simulink model "GFL_GFM"  (R2024b)
settings: Solver=FixedStepAuto  StartTime=0.0  StopTime=1.2  FixedStep=1E-6  RelTol=1e-3
InitFcn:
  | %电网阻抗参数-------------------------------
  | Rg=0.000008; Lg=0.4e-3;
  | Sn=2000000;
  | k=0.6;
  | %分配比例,在这里设置分配比例，GFL：GFM=k:(1-k)
  | PGFL=Sn*k;PGFM=Sn*(1-k);
  | 
  | %GFL参数------------------------------------
  | L_GFL=70e-6;  C_GFL=80e-6; R_GFL=0.2;
  | R1=0;L1=2e-4;
  | Ppll=0.8;Ipll=200;
  | Pp_GFL=0.001;Ip_GFL=0.14;
  | %电流环参数
  | Pp=0.0002;Ip=0.06;Max=2000;
  | Pp2=0.0002;Ip2=0.0008;Max2=200;
  | Pi_GFL=5;Ii_GFL=500;
  | 
  | %GFM参数------------------------------------
  | L_GFM=35e-6; R_GFM=0; C_GFM=150e-6;
  | R2=0;L2=1e-4;
  | %功率环
  | J=7.8; D=1200; Kf=300;
  | Kv=200; Ku=120;
  | %电压电流内环
  | Pv_GFM=66;Iv_GFM=800;
  | Pi_GFM=10;Ii_GFM=100;
model workspace (MAT data in the model file):
  uniqueStringPll_745 = '81_4724'
libraries: spsSeriesRLCBranchLib x12, slpidlib x11, spsabctodq0Lib x7, spsThreePhaseVIMeasurementLib x4, spsGroundLib x3, spsThreePhaseSeriesRLCBranchLib x3, spsThreePhaseTransformerTwoWindingsLib x3, spsDCVoltageSourceLib x2, spsPWMGenerator3LevelLib x2, spsdq0toabcLib x2, spsThreeLevelBridgeLib x2, spsPLL3phLib x1
(part 1 of 2)
settings Model: Creator=Simulink  LastModifiedBy=SESA504213
settings SolverCC: AlgebraicLoopSolver=TrustRegion
settings DataIOCC: ReturnWorkspaceOutputs=off
settings DebuggingCC: UnconnectedInputMsg=warning  UnconnectedOutputMsg=warning  UnconnectedLineMsg=warning  ArithmeticOperatorsInVariantConditions=warning
settings ModelReferenceCC: EnableRefExpFcnMdlSchedulingChecks=on
settings SFSimCC: CustomCodeUndefinedFunction=UseInterfaceOnly
settings RTWCC: GPUComputeCapability=3.5
settings SimscapeCC: SimscapeLogType=all  SimscapeLogLimitData=off

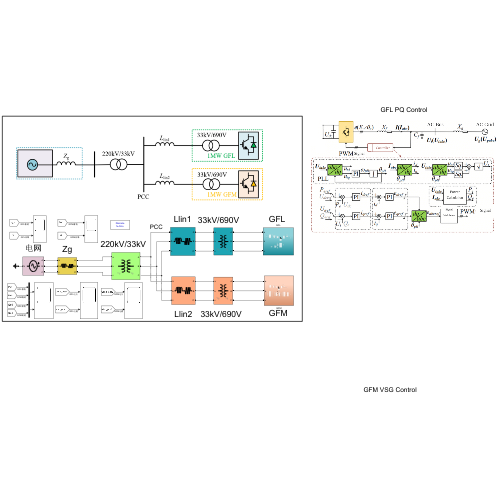
[thumbnail: Simulink's stored preview of the top-level diagram]
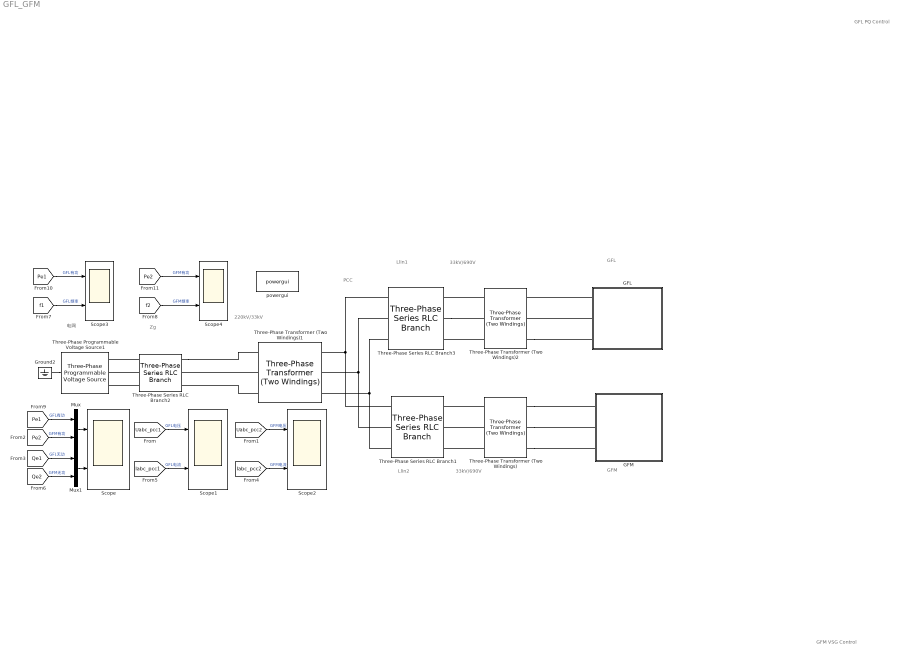
== system GFL_GFM ==
  note: GFL PQ Control
  note: Llin1
  note: PCC
  note: 220kV/33kV
  note: 电网
  note: Zg
  note: Llin2
  note: 33kV/690V
  note: 33kV/690V
  note: GFL
  note: GFM
  note: GFM VSG Control
  GFL : Subsystem
  GFM : Subsystem
  Ground2 : spsGroundLib/Ground  LConnTagsString=a
  Mux : Mux  Inputs=2
  Mux1 : Mux  Inputs=2
  Scope{,1..4} (5 alike) : Scope  NumInputPorts=2
  Three-Phase Programmable Voltage Source1 : spsThreePhaseProgrammableVoltageSourceLib/Three-Phase Programmable Voltage Source  PositiveSequence=[220e3 0 50]  VariationEntity=Frequency  VariationType=Step  VariationTypeAlt=Step  VariationStep=-0.1  VariationRate=10  VariationMagnitude=0.3  VariationFrequency=2  VariationTiming=[0.4 0.8]  VariationPhaseA=off  Amplitudes=[1 0.8 1.2 1.0]  TimeValues=[0 0.1 0.15 0.2]  HarmonicGeneration=off  HarmonicA=[3 0.2 -25 0]  HarmonicB=[2 0.15 35 2]  Timing="[0.05  3]"  BusType=swing  Pref=0  Qref=0  Qmin=-inf  Qmax=inf
  Three-Phase Series RLC Branch1 : spsThreePhaseSeriesRLCBranchLib/Three-Phase Series RLC Branch  LConnTagsString=A|B|C  RConnTagsString=A|B|C  BranchType=RL  Resistance=R2  Inductance=L2  Capacitance=1e-6  Measurements=None
  Three-Phase Series RLC Branch2 : spsThreePhaseSeriesRLCBranchLib/Three-Phase Series RLC Branch  LConnTagsString=A|B|C  RConnTagsString=A|B|C  BranchType=RL  Resistance=Rg*(10e3/690)*(10e3/690)  Inductance=Lg*(10e3/690)*(10e3/690)  Capacitance=1e-6  Measurements=None
  Three-Phase Series RLC Branch3 : spsThreePhaseSeriesRLCBranchLib/Three-Phase Series RLC Branch  LConnTagsString=A|B|C  RConnTagsString=A|B|C  BranchType=RL  Resistance=R1  Inductance=L1  Capacitance=1e-6  Measurements=None
  Three-Phase Transformer (Two Windings) : spsThreePhaseTransformerTwoWindingsLib/Three-Phase Transformer (Two Windings)  Winding1Connection=Yg  Winding2Connection=Yg  CoreType=Three single-phase transformers  SetSaturation=off  Hysteresis=off  DataFile='hysteresis'  SetInitialFlux=off  Measurements=None  UNITS=pu  NominalPower=[ 5e6 , 50 ]  Winding1=[ 690 , 0.002 , 0.08 ]  Winding2=[ 33e3 , 0.002 , 0.08 ]  Rm=500  Lm=500  L0=0.5  Saturation=[ 0,0 ; 0.0024,1.2 ; 1.0,1.52 ]  InitialFluxes=[ 0.8 , -0.8 , 0.7 ]  BreakLoop=off  DiscreteSolver=Trapezoidal iterative  DataType=off  TransfoNumber=1
  Three-Phase Transformer (Two Windings)1 : spsThreePhaseTransformerTwoWindingsLib/Three-Phase Transformer (Two Windings)  Winding1Connection=Yg  Winding2Connection=Yg  CoreType=Three single-phase transformers  SetSaturation=off  Hysteresis=off  DataFile='hysteresis'  SetInitialFlux=off  Measurements=None  UNITS=pu  NominalPower=[ 5e6 , 50 ]  Winding1=[ 33e3 , 0.002 , 0.08 ]  Winding2=[ 220e3 , 0.002 , 0.08 ]  Rm=500  Lm=500  L0=0.5  Saturation=[ 0,0 ; 0.0024,1.2 ; 1.0,1.52 ]  InitialFluxes=[ 0.8 , -0.8 , 0.7 ]  BreakLoop=off  DiscreteSolver=Trapezoidal iterative  DataType=off  TransfoNumber=1
  Three-Phase Transformer (Two Windings)2 : spsThreePhaseTransformerTwoWindingsLib/Three-Phase Transformer (Two Windings)  Winding1Connection=Yg  Winding2Connection=Yg  CoreType=Three single-phase transformers  SetSaturation=off  Hysteresis=off  DataFile='hysteresis'  SetInitialFlux=off  Measurements=None  UNITS=pu  NominalPower=[ 5e6 , 60 ]  Winding1=[ 690 , 0.002 , 0.08 ]  Winding2=[33e3 , 0.002 , 0.08 ]  Rm=500  Lm=500  L0=0.5  Saturation=[ 0,0 ; 0.0024,1.2 ; 1.0,1.52 ]  InitialFluxes=[ 0.8 , -0.8 , 0.7 ]  BreakLoop=off  DiscreteSolver=Trapezoidal iterative  DataType=off  TransfoNumber=1
  powergui : spspowerguiLib/powergui  Priority=1  SimulationMode=Discrete  SampleTime=1E-6  frequency=60  Iterations=50  frequencyindice=0  Pbase=100e6  ErrMax=1e-4  UnitsV=kV  UnitsW=MW  buscounter=0  FunctionMessages=off  echomessages=off  EnableUseOfTLC=off  CurrentSourceSwitches=off  DisableSnubberDevices=off  DisableRonSwitches=off  DisableVfSwitches=off  DisplayEquations=off  AutomaticDiscreteSolvers=off  SolverType=Tustin/Backward Euler (TBE)  Interpol=off  ExternalGateDelay=off  methode=off  Ts=100  x0status=blocks  SPID=off  SwTol=0  HookPort=off  NonlinearTolerance=1e-4  nMaxIteration=100  ContinueOnMaxIteration=off  RestoreLinks=warning  ResistiveCurrentMeasurement=off  Frange=[0:2:500]  Ylog=off  Xlog=on  ShowGrid=off  save=off  variable=ZData  structure=ScopeData1  ZoomFFT=off  StartTime=0.0  cycles=1  DisplayStyle=1  fundamental=60  FreqAxis=off  MaxFrequency=1000  frequencyindicesteady=1  RmsSteady=1  display=off
  wires:
  [Qe1] -> Mux1/1  "GFL无功"
  [Qe2] -> Mux1/2  "GFM无功"
  Mux/1 -> Scope/1
  [Pe2] -> Mux/2  "GFM有功"
  Mux1/1 -> Scope/2
  [Pe1] -> Mux/1  "GFL有功"
  [Uabc_pcc1] -> Scope1/1  "GFL电压"
  [Iabc_pcc1] -> Scope1/2  "GFL电流"
  [Uabc_pcc2] -> Scope2/1  "GFM电压"
  [Iabc_pcc2] -> Scope2/2  "GFM电流"
  [Pe1] -> Scope3/1  "GFL有功"
  [f1] -> Scope3/2  "GFL频率"
  [Pe2] -> Scope4/1  "GFM有功"
  [f2] -> Scope4/2  "GFM频率"
  connections:
  Three-Phase Transformer (Two Windings)/RConn3 -- Three-Phase Series RLC Branch1/LConn3
  Three-Phase Transformer (Two Windings)/RConn1 -- Three-Phase Series RLC Branch1/LConn1
  Three-Phase Transformer (Two Windings)/RConn2 -- Three-Phase Series RLC Branch1/LConn2
  Ground2/LConn1 -- Three-Phase Programmable Voltage Source1/LConn1
  Three-Phase Transformer (Two Windings)/LConn1 -- GFM/RConn1
  Three-Phase Transformer (Two Windings)/LConn2 -- GFM/RConn2
  Three-Phase Transformer (Two Windings)/LConn3 -- GFM/RConn3
  Three-Phase Series RLC Branch3/RConn2 -- Three-Phase Series RLC Branch1/RConn2 -- Three-Phase Transformer (Two Windings)1/LConn2
  Three-Phase Series RLC Branch3/RConn1 -- Three-Phase Series RLC Branch1/RConn1 -- Three-Phase Transformer (Two Windings)1/LConn1
  Three-Phase Series RLC Branch3/RConn3 -- Three-Phase Series RLC Branch1/RConn3 -- Three-Phase Transformer (Two Windings)1/LConn3
  Three-Phase Transformer (Two Windings)1/RConn2 -- Three-Phase Series RLC Branch2/LConn2
  Three-Phase Series RLC Branch2/LConn1 -- Three-Phase Transformer (Two Windings)1/RConn1
  Three-Phase Transformer (Two Windings)1/RConn3 -- Three-Phase Series RLC Branch2/LConn3
  Three-Phase Series RLC Branch2/RConn1 -- Three-Phase Programmable Voltage Source1/RConn1
  Three-Phase Series RLC Branch2/RConn2 -- Three-Phase Programmable Voltage Source1/RConn2
  Three-Phase Series RLC Branch2/RConn3 -- Three-Phase Programmable Voltage Source1/RConn3
  Three-Phase Transformer (Two Windings)2/LConn3 -- GFL/RConn3
  Three-Phase Transformer (Two Windings)2/RConn1 -- Three-Phase Series RLC Branch3/LConn1
  GFL/RConn2 -- Three-Phase Transformer (Two Windings)2/LConn2
  Three-Phase Series RLC Branch3/LConn2 -- Three-Phase Transformer (Two Windings)2/RConn2
  Three-Phase Transformer (Two Windings)2/RConn3 -- Three-Phase Series RLC Branch3/LConn3
  GFL/RConn1 -- Three-Phase Transformer (Two Windings)2/LConn1

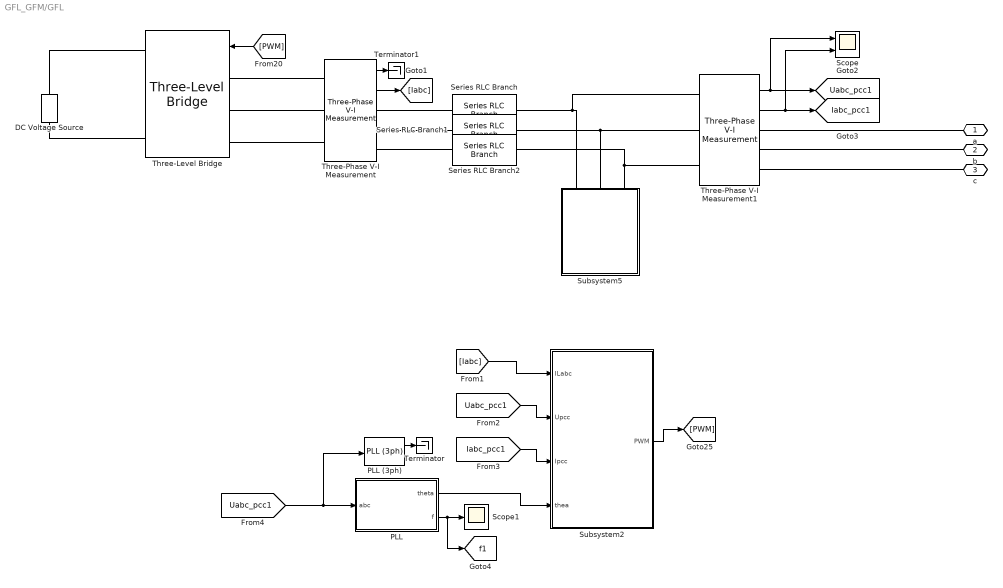
== system GFL_GFM/GFL ==
  DC Voltage Source : spsDCVoltageSourceLib/DC Voltage Source  Amplitude=1500  Measurements=None
  PLL : Subsystem
  PLL (3ph) : spsPLL3phLib/PLL (3ph)  Fmin=45  Par_Init=[0, 50]  ParK=[180, 3200, 1]  TcD=1e-4  MaxRateChangeFreq=12  FilterCutOffFreq=25  Ts=0  AGC=on
  Scope : Scope  NumInputPorts=2
  Scope1 : Scope
  Series RLC Branch : spsSeriesRLCBranchLib/Series RLC Branch  LConnTagsString=__new0  RConnTagsString=__new0  BranchType=L  Resistance=0  Inductance=L_GFL  SetiL0=off  InitialCurrent=0  Capacitance=1e-6  Setx0=off  InitialVoltage=0  Measurements=Branch voltage
  Series RLC Branch1 : spsSeriesRLCBranchLib/Series RLC Branch  LConnTagsString=__new0  RConnTagsString=__new0  BranchType=L  Resistance=0  Inductance=L_GFL  SetiL0=off  InitialCurrent=0  Capacitance=1e-6  Setx0=off  InitialVoltage=0  Measurements=Branch voltage
  Series RLC Branch2 : spsSeriesRLCBranchLib/Series RLC Branch  LConnTagsString=__new0  RConnTagsString=__new0  BranchType=L  Resistance=0  Inductance=L_GFL  SetiL0=off  InitialCurrent=0  Capacitance=1e-6  Setx0=off  InitialVoltage=0  Measurements=Branch voltage
  Subsystem2 : Subsystem
  Subsystem5 : Subsystem
  Terminator : Terminator
  Terminator1 : Terminator
  Three-Level Bridge : spsThreeLevelBridgeLib/Three-Level Bridge  Arms=3  SnubberResistance=1e5  SbubberCapacitance=inf  Device=IGBT / Diodes  Ron=1e-3  ForwardVoltages="[  0  0  ]"  Measurements=None
      settings: LibrarySourceBlock=sps_lib/Power Electronics/Three-Level Bridge
  Three-Phase V-I Measurement : spsThreePhaseVIMeasurementLib/Three-Phase V-I Measurement  VoltageMeasurement=phase-to-ground  SetLabelV=off  LabelV=Vabc  Vpu=off  VpuLL=off  CurrentMeasurement=yes  SetLabelI=off  LabelI=Iabc  Ipu=off  Pbase=100e6  Vbase=500e3  OutputType=Complex  PhasorSimulation=off  PSBequivalent=0
  Three-Phase V-I Measurement1 : spsThreePhaseVIMeasurementLib/Three-Phase V-I Measurement  VoltageMeasurement=phase-to-ground  SetLabelV=off  LabelV=Vabc  Vpu=off  VpuLL=off  CurrentMeasurement=yes  SetLabelI=off  LabelI=Iabc  Ipu=off  Pbase=100e6  Vbase=500e3  OutputType=Complex  PhasorSimulation=off  PSBequivalent=0
  a : PMIOPort  Side=Right
  b : PMIOPort  Port=2  Side=Right
  c : PMIOPort  Port=3  Side=Right
  tag scope: Iabc_pcc1=global, Uabc_pcc1=global, f1=global
  wires:
  Three-Phase V-I Measurement1/2 -> Scope/2, [Iabc_pcc1]
  [PWM] -> Three-Level Bridge/1
  Three-Phase V-I Measurement/2 -> [Iabc]
  PLL (3ph)/1 -> Terminator/1
  Three-Phase V-I Measurement1/1 -> Scope/1, [Uabc_pcc1]
  Three-Phase V-I Measurement/1 -> Terminator1/1
  [Iabc_pcc1] -> Subsystem2/3(Ipcc)
  [Uabc_pcc1] -> Subsystem2/2(Upcc)
  [Iabc] -> Subsystem2/1(ILabc)
  Subsystem2/1(PWM) -> [PWM]
  [Uabc_pcc1] -> PLL (3ph)/1, PLL/1(abc)
  PLL/1(theta) -> Subsystem2/4(thea)
  PLL/2(f) -> [f1], Scope1/1
  connections:
  Three-Phase V-I Measurement/LConn3 -- Three-Level Bridge/LConn3
  Series RLC Branch1/RConn1 -- Three-Phase V-I Measurement1/LConn2 -- Subsystem5/LConn2
  Series RLC Branch/RConn1 -- Subsystem5/LConn1 -- Three-Phase V-I Measurement1/LConn1
  Three-Phase V-I Measurement/RConn3 -- Series RLC Branch2/LConn1
  Three-Level Bridge/LConn2 -- Three-Phase V-I Measurement/LConn2
  Three-Phase V-I Measurement/LConn1 -- Three-Level Bridge/LConn1
  Three-Phase V-I Measurement/RConn2 -- Series RLC Branch1/LConn1
  Three-Level Bridge/RConn1 -- DC Voltage Source/RConn1
  DC Voltage Source/LConn1 -- Three-Level Bridge/RConn3
  Series RLC Branch/LConn1 -- Three-Phase V-I Measurement/RConn1
  Series RLC Branch2/RConn1 -- Subsystem5/LConn3 -- Three-Phase V-I Measurement1/LConn3
  a/RConn1 -- Three-Phase V-I Measurement1/RConn1
  Three-Phase V-I Measurement1/RConn2 -- b/RConn1
  c/RConn1 -- Three-Phase V-I Measurement1/RConn3

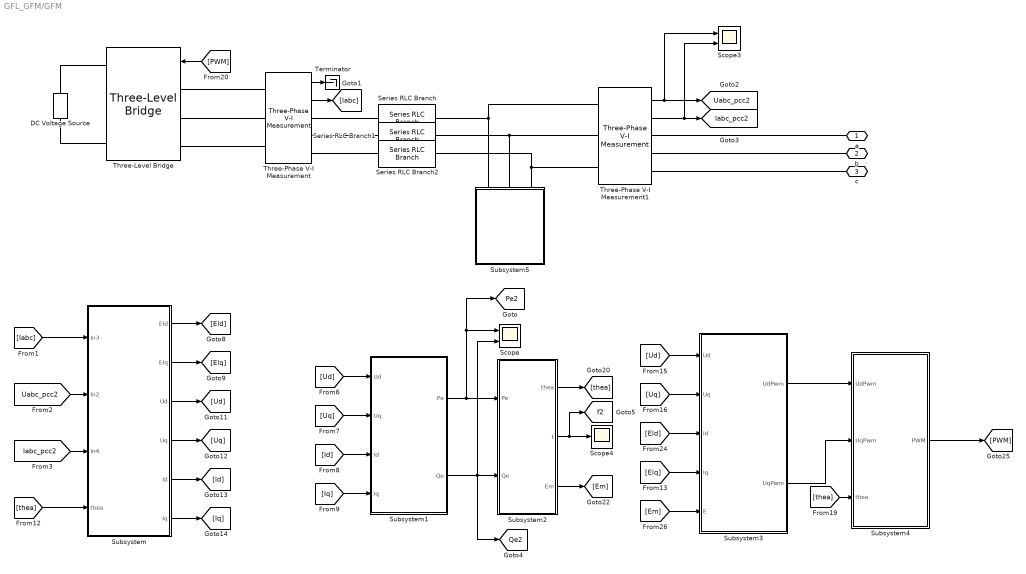
== system GFL_GFM/GFM ==
  DC Voltage Source : spsDCVoltageSourceLib/DC Voltage Source  Amplitude=1500  Measurements=None
  Scope : Scope  NumInputPorts=2
  Scope3 : Scope  NumInputPorts=2
  Scope4 : Scope
  Series RLC Branch : spsSeriesRLCBranchLib/Series RLC Branch  LConnTagsString=__new0  RConnTagsString=__new0  BranchType=L  Resistance=0  Inductance=L_GFM  SetiL0=off  InitialCurrent=0  Capacitance=1e-6  Setx0=off  InitialVoltage=0  Measurements=Branch voltage
  Series RLC Branch1 : spsSeriesRLCBranchLib/Series RLC Branch  LConnTagsString=__new0  RConnTagsString=__new0  BranchType=L  Resistance=0  Inductance=L_GFM  SetiL0=off  InitialCurrent=0  Capacitance=1e-6  Setx0=off  InitialVoltage=0  Measurements=Branch voltage
  Series RLC Branch2 : spsSeriesRLCBranchLib/Series RLC Branch  LConnTagsString=__new0  RConnTagsString=__new0  BranchType=L  Resistance=0  Inductance=L_GFM  SetiL0=off  InitialCurrent=0  Capacitance=1e-6  Setx0=off  InitialVoltage=0  Measurements=Branch voltage
  Subsystem : Subsystem
  Subsystem1 : Subsystem
  Subsystem2 : Subsystem
  Subsystem3 : Subsystem
  Subsystem4 : Subsystem
  Subsystem5 : Subsystem
  Terminator : Terminator
  Three-Level Bridge : spsThreeLevelBridgeLib/Three-Level Bridge  Arms=3  SnubberResistance=1e5  SbubberCapacitance=inf  Device=IGBT / Diodes  Ron=1e-3  ForwardVoltages="[  0  0  ]"  Measurements=None
      settings: LibrarySourceBlock=sps_lib/Power Electronics/Three-Level Bridge
  Three-Phase V-I Measurement : spsThreePhaseVIMeasurementLib/Three-Phase V-I Measurement  VoltageMeasurement=phase-to-ground  SetLabelV=off  LabelV=Vabc  Vpu=off  VpuLL=off  CurrentMeasurement=yes  SetLabelI=off  LabelI=Iabc  Ipu=off  Pbase=100e6  Vbase=500e3  OutputType=Complex  PhasorSimulation=off  PSBequivalent=0
  Three-Phase V-I Measurement1 : spsThreePhaseVIMeasurementLib/Three-Phase V-I Measurement  VoltageMeasurement=phase-to-ground  SetLabelV=off  LabelV=Vabc  Vpu=off  VpuLL=off  CurrentMeasurement=yes  SetLabelI=off  LabelI=Iabc  Ipu=off  Pbase=100e6  Vbase=500e3  OutputType=Complex  PhasorSimulation=off  PSBequivalent=0
  a : PMIOPort  Side=Right
  b : PMIOPort  Port=2  Side=Right
  c : PMIOPort  Port=3  Side=Right
  tag scope: Iabc_pcc2=global, Pe2=global, Qe2=global, Uabc_pcc2=global, f2=global
  wires:
  Three-Phase V-I Measurement1/2 -> Scope3/2, [Iabc_pcc2]
  Three-Phase V-I Measurement1/1 -> Scope3/1, [Uabc_pcc2]
  Three-Phase V-I Measurement/2 -> [Iabc]
  [PWM] -> Three-Level Bridge/1
  Three-Phase V-I Measurement/1 -> Terminator/1
  Subsystem4/1(PWM) -> [PWM]
  [Elq] -> Subsystem3/4(Iq)
  Subsystem2/3(Em) -> [Em]
  [Id] -> Subsystem1/3(Id)
  [Uabc_pcc2] -> Subsystem/2(In2)
  Subsystem/5(Id) -> [Id]
  [Uq] -> Subsystem3/2(Uq)
  [thea] -> Subsystem/4(thea)
  [Ud] -> Subsystem3/1(Ud)
  Subsystem/1(EId) -> [Eld]
  [Eld] -> Subsystem3/3(Id)
  [Em] -> Subsystem3/5(E)
  Subsystem3/2(UqPwm) -> Subsystem4/2(UqPwm)
  Subsystem3/1(UdPwm) -> Subsystem4/1(UdPwm)
  Subsystem2/2(f) -> [f2], Scope4/1
  Subsystem1/2(Qe) -> [Qe2], Scope/2, Subsystem2/2(Qe)
  [Iabc] -> Subsystem/1(In3)
  Subsystem1/1(Pe) -> [Pe2], Scope/1, Subsystem2/1(Pe)
  Subsystem2/1(thea) -> [thea]
  [thea] -> Subsystem4/3(thea)
  [Iq] -> Subsystem1/4(Iq)
  Subsystem/3(Ud) -> [Ud]
  Subsystem/2(EIq) -> [Elq]
  Subsystem/6(Iq) -> [Iq]
  [Uq] -> Subsystem1/2(Uq)
  Subsystem/4(Uq) -> [Uq]
  [Iabc_pcc2] -> Subsystem/3(In4)
  [Ud] -> Subsystem1/1(Ud)
  connections:
  Series RLC Branch/LConn1 -- Three-Phase V-I Measurement/RConn1
  a/RConn1 -- Three-Phase V-I Measurement1/RConn1
  Three-Phase V-I Measurement/RConn3 -- Series RLC Branch2/LConn1
  Three-Phase V-I Measurement/LConn3 -- Three-Level Bridge/LConn3
  Series RLC Branch2/RConn1 -- Subsystem5/LConn3 -- Three-Phase V-I Measurement1/LConn3
  Series RLC Branch1/RConn1 -- Three-Phase V-I Measurement1/LConn2 -- Subsystem5/LConn2
  b/RConn1 -- Three-Phase V-I Measurement1/RConn2
  Series RLC Branch/RConn1 -- Subsystem5/LConn1 -- Three-Phase V-I Measurement1/LConn1
  Three-Level Bridge/LConn2 -- Three-Phase V-I Measurement/LConn2
  Three-Level Bridge/RConn1 -- DC Voltage Source/RConn1
  DC Voltage Source/LConn1 -- Three-Level Bridge/RConn3
  Three-Phase V-I Measurement/RConn2 -- Series RLC Branch1/LConn1
  Three-Phase V-I Measurement/LConn1 -- Three-Level Bridge/LConn1
  c/RConn1 -- Three-Phase V-I Measurement1/RConn3

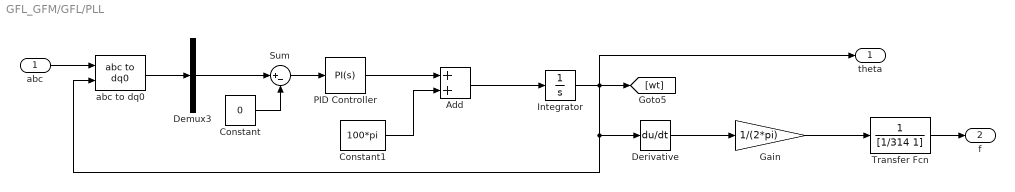
== system GFL_GFM/GFL/PLL ==
  abc : Inport
  Add : Sum
  Constant : Constant  Value=0
  Constant1 : Constant  Value=100*pi
  Demux3 : Demux  Outputs=3
  Derivative : Derivative
  Gain : Gain  Gain=1/(2*pi)
  Integrator : Integrator
  PID Controller : slpidlib/PID Controller  Controller=PI  Form=Parallel  TimeDomain=Continuous-time  UseExternalTs=off  SampleTime=-1  IntegratorMethod=Forward Euler  FilterMethod=Forward Euler  ControllerParametersSource=internal  P=Ppll  I=Ipll  UseKiTs=off  D=0  UseExternalDerivativeSource=off  N=100  UseFilter=on  TunerSelectOption=Transfer Function Based (PID Tuner App)  InitialConditionSource=internal  InitialConditionForIntegrator=0  InitialConditionForFilter=0  DifferentiatorICPrevScaledInput=0  ExternalReset=none  TrackingMode=off  Kt=1  LimitOutput=off  SatLimitsSource=internal  UpperSaturationLimit=inf  LowerSaturationLimit=-inf  LinearizeAsGain=on  AntiWindupMode=none  Kb=1  LimitIntegrator=off  UpperIntegratorSaturationLimit=inf  LowerIntegratorSaturationLimit=-inf  POutMin=[]  POutMax=[]  IOutMin=[]  IOutMax=[]  DOutMin=[]  DOutMax=[]  NOutMin=[]  NOutMax=[]  SumOutMin=[]  SumOutMax=[]  SaturationOutMin=[]  SaturationOutMax=[]  PParamMin=[]  PParamMax=[]  IParamMin=[]  IParamMax=[]  DParamMin=[]  DParamMax=[]  NParamMin=[]  NParamMax=[]  KbParamMin=[]  KbParamMax=[]  KtParamMin=[]  KtParamMax=[]  KbOutMin=[]  KbOutMax=[]  KtOutMin=[]  KtOutMax=[]  IntegratorOutMin=[]  IntegratorOutMax=[]  FilterOutMin=[]  FilterOutMax=[]  SumI1OutMin=[]  SumI1OutMax=[]  SumI2OutMin=[]  SumI2OutMax=[]  SumI3OutMin=[]  SumI3OutMax=[]  SumI4OutMin=[]  SumI4OutMax=[]  SumDOutMin=[]  SumDOutMax=[]  DifferentiatorOutMin=[]  DifferentiatorOutMax=[]  FilterDiffOutCoefMin=[]  FilterDiffOutCoefMax=[]  ReciprocalOutMin=[]  ReciprocalOutMax=[]  SumDenOutMin=[]  SumDenOutMax=[]  SumNumOutMin=[]  SumNumOutMax=[]  DivideOutMin=[]  DivideOutMax=[]  UdiffTsProdOutMin=[]  UdiffTsProdOutMax=[]  NTsProdOutMin=[]  NTsProdOutMax=[]  UintegralTsProdOutMin=[]  UintegralTsProdOutMax=[]  UngainTsProdOutMin=[]  UngainTsProdOutMax=[]  ClampingZeroOutDataTypeStr=Inherit: Inherit via back propagation  ClampingZeroOutMin=[]  ClampingZeroOutMax=[]  FilterDenConstantOutDataTypeStr=Inherit: Inherit via back propagation  FilterDenConstantOutMin=[]  FilterDenConstantOutMax=[]  PCopyOutDataTypeStr=Inherit: Inherit via back propagation  PCopyOutMin=[]  PCopyOutMax=[]  NCopyOutDataTypeStr=Inherit: Inherit via back propagation  NCopyOutMin=[]  NCopyOutMax=[]  IntegratorContinuousStateAttributes=''  IntegratorStateMustResolveToSignalObject=off  IntegratorRTWStateStorageClass=Auto  FilterContinuousStateAttributes=''  FilterStateMustResolveToSignalObject=off  FilterRTWStateStorageClass=Auto  ParallelPVariant=InternalParameters  IdealPVariant=Disabled  IVariant=InternalParameters  DVariant=Disabled  IntegratorVariant=Continuous  SatVariant=Disabled  AWVariant=Passthrough  PCopyVariant=Disabled  TRVariant=Disabled  FdbkBlocksVariant=Forward  IdealPFdbkVariant=Disabled  SatFdbkVariant=Disabled  DerivativeFilterVariant=Disabled  NVariant=Disabled  NCopyVariant=Disabled_SignalSpec  FilterICVariant=Disabled  IntegratorICVariant=InternalICs  ExternalResetVariant=Disabled  TRSumVariant=Passthrough  SumFdbkVariant=Disabled  SumVariant=Sum_PI  TsampFilterVariant=InternalTs  TsampNgainVariant=Passthrough  TsampIntegralVariant=Disabled_SignalSpec  ExternalSaturationOutDataTypeStr=Inherit: Same as second input  DerivativeSourceVariant=Disabled  PreIntVariant=InternalPreInt
  Sum : Sum  Inputs=|+-
  Transfer Fcn : TransferFcn  Denominator=[1/314 1]
  abc to dq0 : spsabctodq0Lib/abc to dq0  Alignment=90 degrees behind phase A axis
  theta : Outport
  f : Outport  Port=2
  wires:
  Demux3/2 -> Sum/1
  Integrator/1 -> theta/1, Derivative/1, abc to dq0/2, [wt]
  abc/1 -> abc to dq0/1
  abc to dq0/1 -> Demux3/1
  Sum/1 -> PID Controller/1
  Constant/1 -> Sum/2
  Gain/1 -> Transfer Fcn/1
  Derivative/1 -> Gain/1
  Constant1/1 -> Add/2
  Add/1 -> Integrator/1
  PID Controller/1 -> Add/1
  Transfer Fcn/1 -> f/1

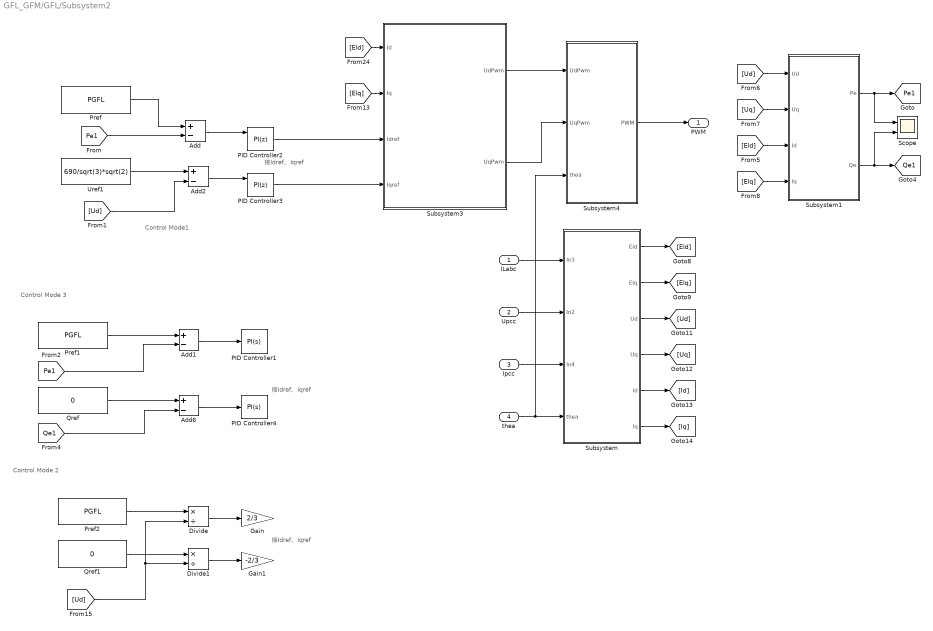
== system GFL_GFM/GFL/Subsystem2 ==
  note: 接Idref、Iqref
  note: Control Mode 3
  note: 接Idref、Iqref
  note: Control Mode 2
  note: Control Mode1
  note: 接Idref、Iqref
  ILabc : Inport
  Upcc : Inport  Port=2
  Ipcc : Inport  Port=3
  thea : Inport  Port=4
  Add{,1..2,6} (4 alike) : Sum  Inputs=+-
  Divide : Product  Inputs=*/
  Divide1 : Product  Inputs=*/
  Gain : Gain  Gain=2/3
  Gain1 : Gain  Gain=-2/3
  PID Controller1 : slpidlib/PID Controller  Controller=PI  Form=Parallel  TimeDomain=Continuous-time  UseExternalTs=off  SampleTime=-1  IntegratorMethod=Forward Euler  FilterMethod=Forward Euler  ControllerParametersSource=internal  P=Pp  I=Ip  UseKiTs=off  D=0  UseExternalDerivativeSource=off  N=100  UseFilter=on  TunerSelectOption=Transfer Function Based (PID Tuner App)  InitialConditionSource=internal  InitialConditionForIntegrator=0  InitialConditionForFilter=0  DifferentiatorICPrevScaledInput=0  ExternalReset=none  TrackingMode=off  Kt=1  LimitOutput=on  SatLimitsSource=internal  UpperSaturationLimit=Max  LowerSaturationLimit=-Max  LinearizeAsGain=on  AntiWindupMode=none  Kb=1  LimitIntegrator=off  UpperIntegratorSaturationLimit=inf  LowerIntegratorSaturationLimit=-inf  POutMin=[]  POutMax=[]  IOutMin=[]  IOutMax=[]  DOutMin=[]  DOutMax=[]  NOutMin=[]  NOutMax=[]  SumOutMin=[]  SumOutMax=[]  SaturationOutMin=[]  SaturationOutMax=[]  PParamMin=[]  PParamMax=[]  IParamMin=[]  IParamMax=[]  DParamMin=[]  DParamMax=[]  NParamMin=[]  NParamMax=[]  KbParamMin=[]  KbParamMax=[]  KtParamMin=[]  KtParamMax=[]  KbOutMin=[]  KbOutMax=[]  KtOutMin=[]  KtOutMax=[]  IntegratorOutMin=[]  IntegratorOutMax=[]  FilterOutMin=[]  FilterOutMax=[]  SumI1OutMin=[]  SumI1OutMax=[]  SumI2OutMin=[]  SumI2OutMax=[]  SumI3OutMin=[]  SumI3OutMax=[]  SumI4OutMin=[]  SumI4OutMax=[]  SumDOutMin=[]  SumDOutMax=[]  DifferentiatorOutMin=[]  DifferentiatorOutMax=[]  FilterDiffOutCoefMin=[]  FilterDiffOutCoefMax=[]  ReciprocalOutMin=[]  ReciprocalOutMax=[]  SumDenOutMin=[]  SumDenOutMax=[]  SumNumOutMin=[]  SumNumOutMax=[]  DivideOutMin=[]  DivideOutMax=[]  UdiffTsProdOutMin=[]  UdiffTsProdOutMax=[]  NTsProdOutMin=[]  NTsProdOutMax=[]  UintegralTsProdOutMin=[]  UintegralTsProdOutMax=[]  UngainTsProdOutMin=[]  UngainTsProdOutMax=[]  ClampingZeroOutDataTypeStr=Inherit: Inherit via back propagation  ClampingZeroOutMin=[]  ClampingZeroOutMax=[]  FilterDenConstantOutDataTypeStr=Inherit: Inherit via back propagation  FilterDenConstantOutMin=[]  FilterDenConstantOutMax=[]  PCopyOutDataTypeStr=Inherit: Inherit via back propagation  PCopyOutMin=[]  PCopyOutMax=[]  NCopyOutDataTypeStr=Inherit: Inherit via back propagation  NCopyOutMin=[]  NCopyOutMax=[]  IntegratorContinuousStateAttributes=''  IntegratorStateMustResolveToSignalObject=off  IntegratorRTWStateStorageClass=Auto  FilterContinuousStateAttributes=''  FilterStateMustResolveToSignalObject=off  FilterRTWStateStorageClass=Auto  ParallelPVariant=InternalParameters  IdealPVariant=Disabled  IVariant=InternalParameters  DVariant=Disabled  IntegratorVariant=Continuous  SatVariant=Enabled  AWVariant=Passthrough  PCopyVariant=Disabled  TRVariant=Disabled  FdbkBlocksVariant=Forward  IdealPFdbkVariant=Disabled  SatFdbkVariant=Disabled  DerivativeFilterVariant=Disabled  NVariant=Disabled  NCopyVariant=Disabled_SignalSpec  FilterICVariant=Disabled  IntegratorICVariant=InternalICs  ExternalResetVariant=Disabled  TRSumVariant=Passthrough  SumFdbkVariant=Disabled  SumVariant=Sum_PI  TsampFilterVariant=InternalTs  TsampNgainVariant=Passthrough  TsampIntegralVariant=Disabled_SignalSpec  ExternalSaturationOutDataTypeStr=Inherit: Same as second input  DerivativeSourceVariant=Disabled  PreIntVariant=InternalPreInt
  PID Controller2 : slpidlib/PID Controller  Controller=PI  Form=Parallel  TimeDomain=Discrete-time  UseExternalTs=off  SampleTime=-1  IntegratorMethod=Forward Euler  FilterMethod=Forward Euler  ControllerParametersSource=internal  P=Pp_GFL  I=Ip_GFL  UseKiTs=off  D=0  UseExternalDerivativeSource=off  N=100  UseFilter=on  TunerSelectOption=Transfer Function Based (PID Tuner App)  InitialConditionSource=internal  InitialConditionForIntegrator=0  InitialConditionForFilter=0  DifferentiatorICPrevScaledInput=0  ExternalReset=rising  TrackingMode=off  Kt=1  LimitOutput=off  SatLimitsSource=internal  UpperSaturationLimit=inf  LowerSaturationLimit=-inf  LinearizeAsGain=on  AntiWindupMode=none  Kb=1  LimitIntegrator=off  UpperIntegratorSaturationLimit=inf  LowerIntegratorSaturationLimit=-inf  POutMin=[]  POutMax=[]  IOutMin=[]  IOutMax=[]  DOutMin=[]  DOutMax=[]  NOutMin=[]  NOutMax=[]  SumOutMin=[]  SumOutMax=[]  SaturationOutMin=[]  SaturationOutMax=[]  PParamMin=[]  PParamMax=[]  IParamMin=[]  IParamMax=[]  DParamMin=[]  DParamMax=[]  NParamMin=[]  NParamMax=[]  KbParamMin=[]  KbParamMax=[]  KtParamMin=[]  KtParamMax=[]  KbOutMin=[]  KbOutMax=[]  KtOutMin=[]  KtOutMax=[]  IntegratorOutMin=[]  IntegratorOutMax=[]  FilterOutMin=[]  FilterOutMax=[]  SumI1OutMin=[]  SumI1OutMax=[]  SumI2OutMin=[]  SumI2OutMax=[]  SumI3OutMin=[]  SumI3OutMax=[]  SumI4OutMin=[]  SumI4OutMax=[]  SumDOutMin=[]  SumDOutMax=[]  DifferentiatorOutMin=[]  DifferentiatorOutMax=[]  FilterDiffOutCoefMin=[]  FilterDiffOutCoefMax=[]  ReciprocalOutMin=[]  ReciprocalOutMax=[]  SumDenOutMin=[]  SumDenOutMax=[]  SumNumOutMin=[]  SumNumOutMax=[]  DivideOutMin=[]  DivideOutMax=[]  UdiffTsProdOutMin=[]  UdiffTsProdOutMax=[]  NTsProdOutMin=[]  NTsProdOutMax=[]  UintegralTsProdOutMin=[]  UintegralTsProdOutMax=[]  UngainTsProdOutMin=[]  UngainTsProdOutMax=[]  ClampingZeroOutDataTypeStr=Inherit: Inherit via back propagation  ClampingZeroOutMin=[]  ClampingZeroOutMax=[]  FilterDenConstantOutDataTypeStr=Inherit: Inherit via back propagation  FilterDenConstantOutMin=[]  FilterDenConstantOutMax=[]  PCopyOutDataTypeStr=Inherit: Inherit via back propagation  PCopyOutMin=[]  PCopyOutMax=[]  NCopyOutDataTypeStr=Inherit: Inherit via back propagation  NCopyOutMin=[]  NCopyOutMax=[]  IntegratorContinuousStateAttributes=''  IntegratorStateMustResolveToSignalObject=off  IntegratorRTWStateStorageClass=Auto  FilterContinuousStateAttributes=''  FilterStateMustResolveToSignalObject=off  FilterRTWStateStorageClass=Auto  ParallelPVariant=InternalParameters  IdealPVariant=Disabled  IVariant=InternalParameters  DVariant=Disabled  IntegratorVariant=Discrete  SatVariant=Disabled  AWVariant=Passthrough  PCopyVariant=Disabled  TRVariant=Disabled  FdbkBlocksVariant=Forward  IdealPFdbkVariant=Disabled  SatFdbkVariant=Disabled  DerivativeFilterVariant=Disabled  NVariant=Disabled  NCopyVariant=Disabled_SignalSpec  FilterICVariant=Disabled  IntegratorICVariant=InternalICs  ExternalResetVariant=ExternalReset  TRSumVariant=Passthrough  SumFdbkVariant=Disabled  SumVariant=Sum_PI  TsampFilterVariant=InternalTs  TsampNgainVariant=Passthrough  TsampIntegralVariant=Disabled_SignalSpec  ExternalSaturationOutDataTypeStr=Inherit: Same as second input  DerivativeSourceVariant=Disabled  PreIntVariant=InternalPreInt
  PID Controller3 : slpidlib/PID Controller  Controller=PI  Form=Parallel  TimeDomain=Discrete-time  UseExternalTs=off  SampleTime=-1  IntegratorMethod=Forward Euler  FilterMethod=Forward Euler  ControllerParametersSource=internal  P=Pp_GFL  I=0  UseKiTs=off  D=0  UseExternalDerivativeSource=off  N=100  UseFilter=on  TunerSelectOption=Transfer Function Based (PID Tuner App)  InitialConditionSource=internal  InitialConditionForIntegrator=0  InitialConditionForFilter=0  DifferentiatorICPrevScaledInput=0  ExternalReset=rising  TrackingMode=off  Kt=1  LimitOutput=off  SatLimitsSource=internal  UpperSaturationLimit=inf  LowerSaturationLimit=-inf  LinearizeAsGain=on  AntiWindupMode=none  Kb=1  LimitIntegrator=off  UpperIntegratorSaturationLimit=inf  LowerIntegratorSaturationLimit=-inf  POutMin=[]  POutMax=[]  IOutMin=[]  IOutMax=[]  DOutMin=[]  DOutMax=[]  NOutMin=[]  NOutMax=[]  SumOutMin=[]  SumOutMax=[]  SaturationOutMin=[]  SaturationOutMax=[]  PParamMin=[]  PParamMax=[]  IParamMin=[]  IParamMax=[]  DParamMin=[]  DParamMax=[]  NParamMin=[]  NParamMax=[]  KbParamMin=[]  KbParamMax=[]  KtParamMin=[]  KtParamMax=[]  KbOutMin=[]  KbOutMax=[]  KtOutMin=[]  KtOutMax=[]  IntegratorOutMin=[]  IntegratorOutMax=[]  FilterOutMin=[]  FilterOutMax=[]  SumI1OutMin=[]  SumI1OutMax=[]  SumI2OutMin=[]  SumI2OutMax=[]  SumI3OutMin=[]  SumI3OutMax=[]  SumI4OutMin=[]  SumI4OutMax=[]  SumDOutMin=[]  SumDOutMax=[]  DifferentiatorOutMin=[]  DifferentiatorOutMax=[]  FilterDiffOutCoefMin=[]  FilterDiffOutCoefMax=[]  ReciprocalOutMin=[]  ReciprocalOutMax=[]  SumDenOutMin=[]  SumDenOutMax=[]  SumNumOutMin=[]  SumNumOutMax=[]  DivideOutMin=[]  DivideOutMax=[]  UdiffTsProdOutMin=[]  UdiffTsProdOutMax=[]  NTsProdOutMin=[]  NTsProdOutMax=[]  UintegralTsProdOutMin=[]  UintegralTsProdOutMax=[]  UngainTsProdOutMin=[]  UngainTsProdOutMax=[]  ClampingZeroOutDataTypeStr=Inherit: Inherit via back propagation  ClampingZeroOutMin=[]  ClampingZeroOutMax=[]  FilterDenConstantOutDataTypeStr=Inherit: Inherit via back propagation  FilterDenConstantOutMin=[]  FilterDenConstantOutMax=[]  PCopyOutDataTypeStr=Inherit: Inherit via back propagation  PCopyOutMin=[]  PCopyOutMax=[]  NCopyOutDataTypeStr=Inherit: Inherit via back propagation  NCopyOutMin=[]  NCopyOutMax=[]  IntegratorContinuousStateAttributes=''  IntegratorStateMustResolveToSignalObject=off  IntegratorRTWStateStorageClass=Auto  FilterContinuousStateAttributes=''  FilterStateMustResolveToSignalObject=off  FilterRTWStateStorageClass=Auto  ParallelPVariant=InternalParameters  IdealPVariant=Disabled  IVariant=InternalParameters  DVariant=Disabled  IntegratorVariant=Discrete  SatVariant=Disabled  AWVariant=Passthrough  PCopyVariant=Disabled  TRVariant=Disabled  FdbkBlocksVariant=Forward  IdealPFdbkVariant=Disabled  SatFdbkVariant=Disabled  DerivativeFilterVariant=Disabled  NVariant=Disabled  NCopyVariant=Disabled_SignalSpec  FilterICVariant=Disabled  IntegratorICVariant=InternalICs  ExternalResetVariant=ExternalReset  TRSumVariant=Passthrough  SumFdbkVariant=Disabled  SumVariant=Sum_PI  TsampFilterVariant=InternalTs  TsampNgainVariant=Passthrough  TsampIntegralVariant=Disabled_SignalSpec  ExternalSaturationOutDataTypeStr=Inherit: Same as second input  DerivativeSourceVariant=Disabled  PreIntVariant=InternalPreInt
  PID Controller4 : slpidlib/PID Controller  Controller=PI  Form=Parallel  TimeDomain=Continuous-time  UseExternalTs=off  SampleTime=-1  IntegratorMethod=Forward Euler  FilterMethod=Forward Euler  ControllerParametersSource=internal  P=Pp2  I=Ip2  UseKiTs=off  D=0  UseExternalDerivativeSource=off  N=100  UseFilter=on  TunerSelectOption=Transfer Function Based (PID Tuner App)  InitialConditionSource=internal  InitialConditionForIntegrator=0  InitialConditionForFilter=0  DifferentiatorICPrevScaledInput=0  ExternalReset=none  TrackingMode=off  Kt=1  LimitOutput=on  SatLimitsSource=internal  UpperSaturationLimit=Max2  LowerSaturationLimit=-Max2  LinearizeAsGain=on  AntiWindupMode=none  Kb=1  LimitIntegrator=off  UpperIntegratorSaturationLimit=inf  LowerIntegratorSaturationLimit=-inf  POutMin=[]  POutMax=[]  IOutMin=[]  IOutMax=[]  DOutMin=[]  DOutMax=[]  NOutMin=[]  NOutMax=[]  SumOutMin=[]  SumOutMax=[]  SaturationOutMin=[]  SaturationOutMax=[]  PParamMin=[]  PParamMax=[]  IParamMin=[]  IParamMax=[]  DParamMin=[]  DParamMax=[]  NParamMin=[]  NParamMax=[]  KbParamMin=[]  KbParamMax=[]  KtParamMin=[]  KtParamMax=[]  KbOutMin=[]  KbOutMax=[]  KtOutMin=[]  KtOutMax=[]  IntegratorOutMin=[]  IntegratorOutMax=[]  FilterOutMin=[]  FilterOutMax=[]  SumI1OutMin=[]  SumI1OutMax=[]  SumI2OutMin=[]  SumI2OutMax=[]  SumI3OutMin=[]  SumI3OutMax=[]  SumI4OutMin=[]  SumI4OutMax=[]  SumDOutMin=[]  SumDOutMax=[]  DifferentiatorOutMin=[]  DifferentiatorOutMax=[]  FilterDiffOutCoefMin=[]  FilterDiffOutCoefMax=[]  ReciprocalOutMin=[]  ReciprocalOutMax=[]  SumDenOutMin=[]  SumDenOutMax=[]  SumNumOutMin=[]  SumNumOutMax=[]  DivideOutMin=[]  DivideOutMax=[]  UdiffTsProdOutMin=[]  UdiffTsProdOutMax=[]  NTsProdOutMin=[]  NTsProdOutMax=[]  UintegralTsProdOutMin=[]  UintegralTsProdOutMax=[]  UngainTsProdOutMin=[]  UngainTsProdOutMax=[]  ClampingZeroOutDataTypeStr=Inherit: Inherit via back propagation  ClampingZeroOutMin=[]  ClampingZeroOutMax=[]  FilterDenConstantOutDataTypeStr=Inherit: Inherit via back propagation  FilterDenConstantOutMin=[]  FilterDenConstantOutMax=[]  PCopyOutDataTypeStr=Inherit: Inherit via back propagation  PCopyOutMin=[]  PCopyOutMax=[]  NCopyOutDataTypeStr=Inherit: Inherit via back propagation  NCopyOutMin=[]  NCopyOutMax=[]  IntegratorContinuousStateAttributes=''  IntegratorStateMustResolveToSignalObject=off  IntegratorRTWStateStorageClass=Auto  FilterContinuousStateAttributes=''  FilterStateMustResolveToSignalObject=off  FilterRTWStateStorageClass=Auto  ParallelPVariant=InternalParameters  IdealPVariant=Disabled  IVariant=InternalParameters  DVariant=Disabled  IntegratorVariant=Continuous  SatVariant=Enabled  AWVariant=Passthrough  PCopyVariant=Disabled  TRVariant=Disabled  FdbkBlocksVariant=Forward  IdealPFdbkVariant=Disabled  SatFdbkVariant=Disabled  DerivativeFilterVariant=Disabled  NVariant=Disabled  NCopyVariant=Disabled_SignalSpec  FilterICVariant=Disabled  IntegratorICVariant=InternalICs  ExternalResetVariant=Disabled  TRSumVariant=Passthrough  SumFdbkVariant=Disabled  SumVariant=Sum_PI  TsampFilterVariant=InternalTs  TsampNgainVariant=Passthrough  TsampIntegralVariant=Disabled_SignalSpec  ExternalSaturationOutDataTypeStr=Inherit: Same as second input  DerivativeSourceVariant=Disabled  PreIntVariant=InternalPreInt
  Pref : Constant  Value=PGFL
  Pref1 : Constant  Value=PGFL
  Pref2 : Constant  Value=PGFL
  Qref : Constant  Value=0
  Qref1 : Constant  Value=0
  Scope : Scope  NumInputPorts=2
  Subsystem : Subsystem
  Subsystem1 : Subsystem
  Subsystem3 : Subsystem
  Subsystem4 : Subsystem
  Uref1 : Constant  Value=690/sqrt(3)*sqrt(2)
  PWM : Outport
  tag scope: Pe1=global, Qe1=global
  wires:
  [Ud] -> Subsystem1/1(Ud)
  [Elq] -> Subsystem1/4(Iq)
  Subsystem/3(Ud) -> [Ud]
  [Eld] -> Subsystem3/1(Id)
  Subsystem1/2(Qe) -> [Qe1], Scope/2
  [Uq] -> Subsystem1/2(Uq)
  [Eld] -> Subsystem1/3(Id)
  Subsystem/5(Id) -> [Id]
  Subsystem1/1(Pe) -> [Pe1], Scope/1
  Ipcc/1 -> Subsystem/3(In4)
  [Elq] -> Subsystem3/2(Iq)
  thea/1 -> Subsystem4/3(thea), Subsystem/4(thea)
  Subsystem3/1(UdPwm) -> Subsystem4/1(UdPwm)
  Subsystem/4(Uq) -> [Uq]
  Subsystem/6(Iq) -> [Iq]
  Subsystem3/2(UqPwm) -> Subsystem4/2(UqPwm)
  Subsystem/1(EId) -> [Eld]
  Subsystem/2(EIq) -> [Elq]
  ILabc/1 -> Subsystem/1(In3)
  Upcc/1 -> Subsystem/2(In2)
  Subsystem4/1(PWM) -> PWM/1
  PID Controller2/1 -> Subsystem3/3(Idref)
  PID Controller3/1 -> Subsystem3/4(Iqref)
  Qref/1 -> Add6/1
  [Qe1] -> Add6/2
  [Pe1] -> Add1/2
  Qref1/1 -> Divide1/1
  Add6/1 -> PID Controller4/1
  [Ud] -> Divide1/2, Divide/2
  Pref2/1 -> Divide/1
  Add1/1 -> PID Controller1/1
  Divide/1 -> Gain/1
  Divide1/1 -> Gain1/1
  Pref1/1 -> Add1/1
  Uref1/1 -> Add2/1
  [Ud] -> Add2/2
  Add2/1 -> PID Controller3/1
  Add/1 -> PID Controller2/1
  [Pe1] -> Add/2
  Pref/1 -> Add/1

== system GFL_GFM/GFL/Subsystem5 ==
  Ground : spsGroundLib/Ground  LConnTagsString=a
  Series RLC Branch4 : spsSeriesRLCBranchLib/Series RLC Branch  LConnTagsString=__new0  RConnTagsString=__new0  BranchType=RC  Resistance=R_GFL  Inductance=1e-3  SetiL0=off  InitialCurrent=0  Capacitance=C_GFL  Setx0=off  InitialVoltage=311  Measurements=None
  Series RLC Branch5 : spsSeriesRLCBranchLib/Series RLC Branch  LConnTagsString=__new0  RConnTagsString=__new0  BranchType=RC  Resistance=R_GFL  Inductance=1e-3  SetiL0=off  InitialCurrent=0  Capacitance=C_GFL  Setx0=off  InitialVoltage=311  Measurements=None
  Series RLC Branch6 : spsSeriesRLCBranchLib/Series RLC Branch  LConnTagsString=__new0  RConnTagsString=__new0  BranchType=RC  Resistance=R_GFL  Inductance=1e-3  SetiL0=off  InitialCurrent=0  Capacitance=C_GFL  Setx0=off  InitialVoltage=311  Measurements=None
  Series RLC Branch1 : PMIOPort  Side=Left
  Series RLC Branch2 : PMIOPort  Port=2  Side=Left
  Series RLC Branch3 : PMIOPort  Port=3  Side=Left
  connections:
  Series RLC Branch4/LConn1 -- Series RLC Branch2/RConn1
  Series RLC Branch5/RConn1 -- Ground/LConn1 -- Series RLC Branch4/RConn1 -- Series RLC Branch6/RConn1
  Series RLC Branch5/LConn1 -- Series RLC Branch1/RConn1
  Series RLC Branch6/LConn1 -- Series RLC Branch3/RConn1

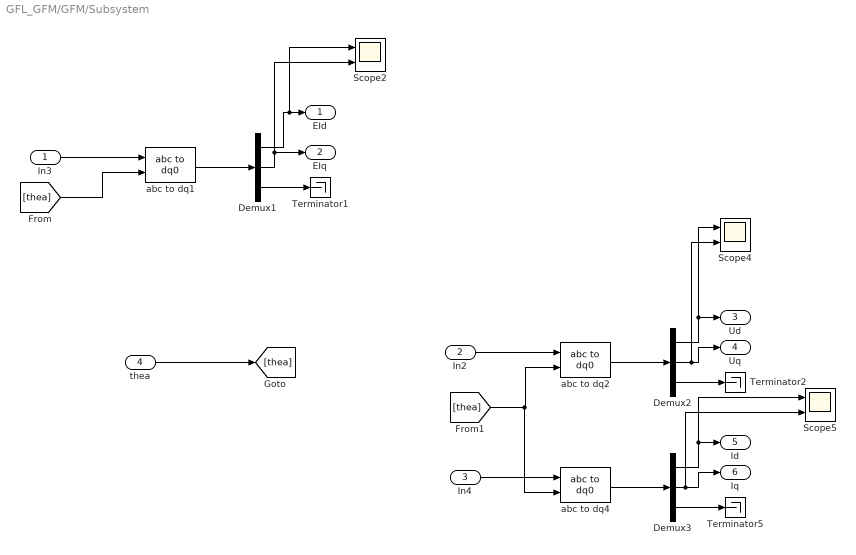
== system GFL_GFM/GFM/Subsystem ==
  In3 : Inport
  In2 : Inport  Port=2
  In4 : Inport  Port=3
  thea : Inport  Port=4
  Demux1 : Demux  Outputs=3
  Demux2 : Demux  Outputs=3
  Demux3 : Demux  Outputs=3
  Scope2 : Scope  NumInputPorts=2
  Scope4 : Scope  NumInputPorts=2
  Scope5 : Scope  NumInputPorts=2
  Terminator1 : Terminator
  Terminator2 : Terminator
  Terminator5 : Terminator
  abc to dq1 : spsabctodq0Lib/abc to dq0  Alignment=90 degrees behind phase A axis
  abc to dq2 : spsabctodq0Lib/abc to dq0  Alignment=90 degrees behind phase A axis
  abc to dq4 : spsabctodq0Lib/abc to dq0  Alignment=90 degrees behind phase A axis
  EId : Outport
  EIq : Outport  Port=2
  Ud : Outport  Port=3
  Uq : Outport  Port=4
  Id : Outport  Port=5
  Iq : Outport  Port=6
  wires:
  In3/1 -> abc to dq1/1
  In2/1 -> abc to dq2/1
  In4/1 -> abc to dq4/1
  abc to dq2/1 -> Demux2/1
  abc to dq4/1 -> Demux3/1
  abc to dq1/1 -> Demux1/1
  Demux2/3 -> Terminator2/1
  Demux3/3 -> Terminator5/1
  Demux1/3 -> Terminator1/1
  Demux1/1 -> Scope2/1, EId/1
  Demux1/2 -> Scope2/2, EIq/1
  Demux2/1 -> Scope4/1, Ud/1
  Demux2/2 -> Scope4/2, Uq/1
  Demux3/1 -> Id/1, Scope5/1
  Demux3/2 -> Scope5/2, Iq/1
  thea/1 -> [thea]
  [thea] -> abc to dq1/2
  [thea] -> abc to dq4/2, abc to dq2/2

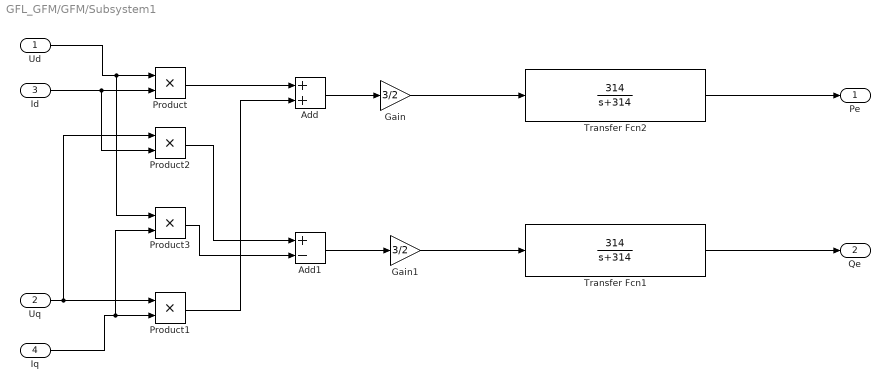
== system GFL_GFM/GFM/Subsystem1 ==
  Ud : Inport
  Uq : Inport  Port=2
  Id : Inport  Port=3
  Iq : Inport  Port=4
  Add : Sum
  Add1 : Sum  Inputs=+-
  Gain : Gain  Gain=3/2
  Gain1 : Gain  Gain=3/2
  Product{,1..3} (4 alike) : Product
  Transfer Fcn1 : TransferFcn  Numerator=[314]  Denominator=[1 314]
  Transfer Fcn2 : TransferFcn  Numerator=[314]  Denominator=[1 314]
  Pe : Outport
  Qe : Outport  Port=2
  wires:
  Ud/1 -> Product3/1, Product/1
  Id/1 -> Product2/2, Product/2
  Uq/1 -> Product2/1, Product1/1
  Iq/1 -> Product1/2, Product3/2
  Add/1 -> Gain/1
  Add1/1 -> Gain1/1
  Product/1 -> Add/1
  Product1/1 -> Add/2
  Product2/1 -> Add1/1
  Product3/1 -> Add1/2
  Gain/1 -> Transfer Fcn2/1
  Gain1/1 -> Transfer Fcn1/1
  Transfer Fcn2/1 -> Pe/1
  Transfer Fcn1/1 -> Qe/1

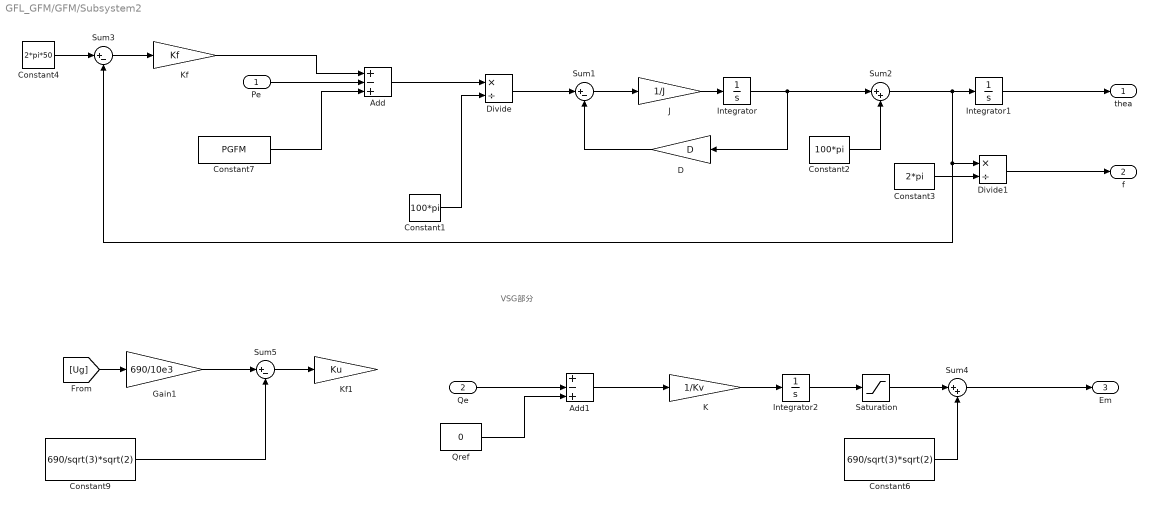
== system GFL_GFM/GFM/Subsystem2 ==
  note: VSG部分
  Pe : Inport
  Qe : Inport  Port=2
  Add : Sum  Inputs=+-+
  Add1 : Sum  Inputs=+-+
  Constant1 : Constant  Value=100*pi
  Constant2 : Constant  Value=100*pi
  Constant3 : Constant  Value=2*pi
  Constant4 : Constant  Value=2*pi*50
  Constant6 : Constant  Value=690/sqrt(3)*sqrt(2)
  Constant7 : Constant  Value=PGFM
  Constant9 : Constant  Value=690/sqrt(3)*sqrt(2)
  D : Gain  Gain=D
  Divide : Product  Inputs=*/
  Divide1 : Product  Inputs=*/
  Gain1 : Gain  Gain=690/10e3
  Integrator : Integrator
  Integrator1 : Integrator
  Integrator2 : Integrator
  J : Gain  Gain=1/J
  K : Gain  Gain=1/Kv
  Kf : Gain  Gain=Kf
  Kf1 : Gain  Gain=Ku
  Qref : Constant  Value=0
  Saturation : Saturate  UpperLimit=100  LowerLimit=-100
  Sum1 : Sum  Inputs=|+-
  Sum2 : Sum  Inputs=|++
  Sum3 : Sum  Inputs=|+-
  Sum4 : Sum  Inputs=|++
  Sum5 : Sum  Inputs=|+-
  thea : Outport
  f : Outport  Port=2
  Em : Outport  Port=3
  wires:
  Pe/1 -> Add/2
  Add/1 -> Divide/1
  Constant1/1 -> Divide/2
  Divide/1 -> Sum1/1
  Sum1/1 -> J/1
  Integrator/1 -> Sum2/1, D/1
  Constant2/1 -> Sum2/2
  D/1 -> Sum1/2
  Sum2/1 -> Integrator1/1, Sum3/2, Divide1/1
  Integrator1/1 -> thea/1
  Divide1/1 -> f/1
  Constant3/1 -> Divide1/2
  Qe/1 -> Add1/2
  Add1/1 -> K/1
  Constant6/1 -> Sum4/2
  Sum4/1 -> Em/1
  J/1 -> Integrator/1
  Sum3/1 -> Kf/1
  Constant4/1 -> Sum3/1
  Qref/1 -> Add1/3
  K/1 -> Integrator2/1
  Saturation/1 -> Sum4/1
  Integrator2/1 -> Saturation/1
  Kf/1 -> Add/1
  [Ug] -> Gain1/1
  Sum5/1 -> Kf1/1
  Constant9/1 -> Sum5/2
  Constant7/1 -> Add/3
  Gain1/1 -> Sum5/1
